simulink model "Question6stepInput_AkankshaMurali"  (R2023b)
settings: Solver=VariableStepAuto  StartTime=0.0  StopTime=10.0  RelTol=1e-3
settings Model: Creator=tina  LastModifiedBy=akank
settings OptimizationCC: ReuseModelBlockBuffer=off

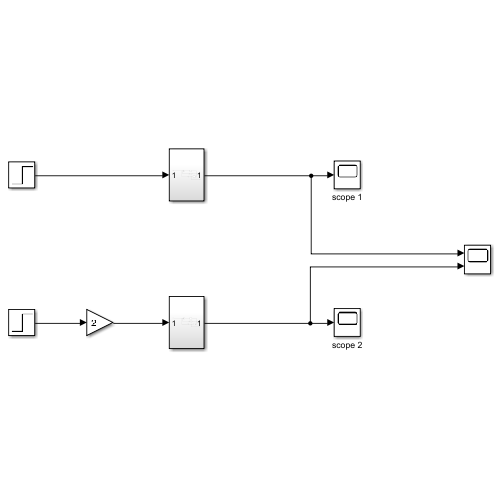
[thumbnail: Simulink's stored preview of the top-level diagram]
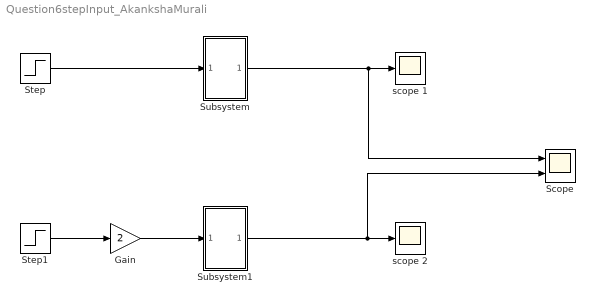
== system Question6stepInput_AkankshaMurali ==
  Gain : Gain  Gain=2
  Scope : Scope  NumInputPorts=2
  Step : Step  SampleTime=0
  Step1 : Step  SampleTime=0
  Subsystem : Subsystem
  Subsystem1 : Subsystem
  scope 1 : Scope
  scope 2 : Scope
  wires:
  Subsystem/1(Out1) -> Scope/1, scope 1/1
  Step/1 -> Subsystem/1(In1)
  Step1/1 -> Gain/1
  Subsystem1/1(Out1) -> Scope/2, scope 2/1
  Gain/1 -> Subsystem1/1(In1)

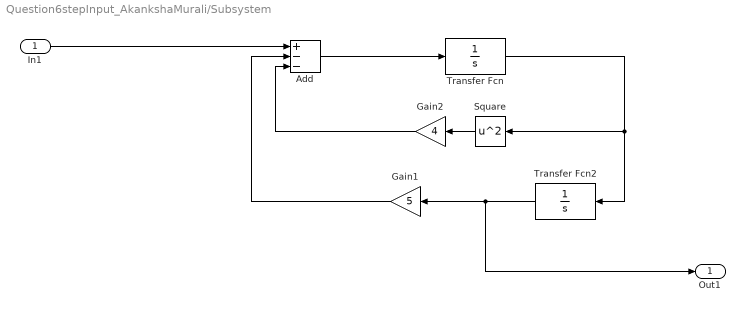
== system Question6stepInput_AkankshaMurali/Subsystem ==
  In1 : Inport
  Add : Sum  Inputs=+--
  Gain1 : Gain  Gain=5
  Gain2 : Gain  Gain=4
  Square : Math  Operator=square  OutputSignalType=real
  Transfer Fcn : TransferFcn  Denominator=[1 0]
  Transfer Fcn2 : TransferFcn  Denominator=[1 0]
  Out1 : Outport
  wires:
  Gain1/1 -> Add/2
  Transfer Fcn2/1 -> Out1/1, Gain1/1
  Square/1 -> Gain2/1
  Gain2/1 -> Add/3
  Add/1 -> Transfer Fcn/1
  In1/1 -> Add/1
  Transfer Fcn/1 -> Square/1, Transfer Fcn2/1

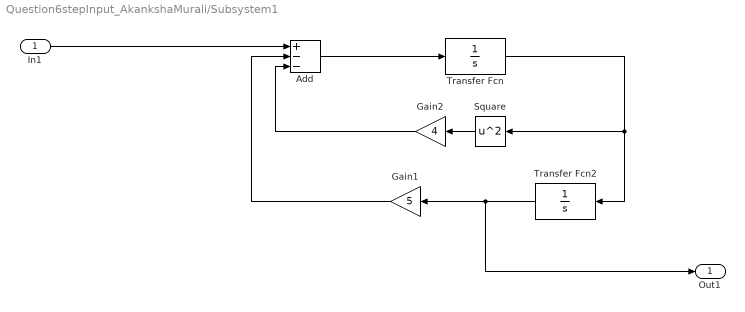
== system Question6stepInput_AkankshaMurali/Subsystem1 ==
  In1 : Inport
  Add : Sum  Inputs=+--
  Gain1 : Gain  Gain=5
  Gain2 : Gain  Gain=4
  Square : Math  Operator=square  OutputSignalType=real
  Transfer Fcn : TransferFcn  Denominator=[1 0]
  Transfer Fcn2 : TransferFcn  Denominator=[1 0]
  Out1 : Outport
  wires:
  Gain1/1 -> Add/2
  Transfer Fcn2/1 -> Out1/1, Gain1/1
  Square/1 -> Gain2/1
  Gain2/1 -> Add/3
  Add/1 -> Transfer Fcn/1
  In1/1 -> Add/1
  Transfer Fcn/1 -> Square/1, Transfer Fcn2/1
